simulink library "inp"  (R2021b)
settings: Solver=VariableStepAuto  StartTime=0.0  StopTime=10.0  RelTol=1e-3
undefined symbols (not defined in the file): C_TASK_5MS_S, FALSE, KINP_AcoreReadyToSlp_flg_ovrdflg, KINP_AcoreReadyToSlp_flg_ovrdval, KINP_AllowMovThd_OTA_enum_ovrdflg, KINP_AllowMovThd_OTA_enum_ovrdval, KINP_APSAngleTarget_Deg_ovrdflg, KINP_APSAngleTarget_Deg_ovrdval, KINP_APSDecReq_mps2_ovrdflg, KINP_APSDecReq_mps2_ovrdval, KINP_APSDecReqA_flg_ovrdflg, KINP_APSDecReqA_flg_ovrdval, KINP_APSDFLL_cm_ovrdflg, KINP_APSDFLL_cm_ovrdval, KINP_APSDFLR_cm_ovrdflg, KINP_APSDFLR_cm_ovrdval, KINP_APSDRLL_cm_ovrdflg, KINP_APSDRLL_cm_ovrdval, KINP_APSDRLR_cm_ovrdflg, KINP_APSDRLR_cm_ovrdval, KINP_APSExitCondition_enum_ovrdflg, KINP_APSExitCondition_enum_ovrdval, KINP_APSHWVer_enum_ovrdflg, KINP_APSHWVer_enum_ovrdval, KINP_APSProgressPCT_pct_ovrdflg, KINP_APSProgressPCT_pct_ovrdval, KINP_APSPwrReq_enum_ovrdflg, KINP_APSPwrReq_enum_ovrdval, KINP_APSReq_enum_ovrdflg, KINP_APSReq_enum_ovrdval, KINP_APSRQDisplay_enum_ovrdflg, KINP_APSRQDisplay_enum_ovrdval, KINP_APSRqEPASCtrl_flg_ovrdflg, KINP_APSRqEPASCtrl_flg_ovrdval, KINP_APSShiftPosnReq_enum_ovrdval, KINP_APSShiftPosnReq_enum_ovrflg, KINP_APSSpeedCMD_kph_ovrdval, KINP_APSSpeedCMD_kph_ovrflg, KINP_APSStaSystem_enum_ovrdflg, KINP_APSStaSystem_enum_ovrdval, KINP_APSSWVer_enum_ovrdflg, KINP_APSSWVer_enum_ovrdval, KINP_APSVMCReqA_flg_ovrdval, KINP_APSVMCReqA_flg_ovrflg, KINP_APSVRqEPASCtrl_flg_ovrdflg, KINP_APSVRqEPASCtrl_flg_ovrdval, KINP_AuxBattVolmV_mV_ovrdflg, KINP_AuxBattVolmV_mV_ovrdval, KINP_BTConnectSta_enum_ovrdflg, KINP_BTConnectSta_enum_ovrdval, KINP_CAASSta_enum_ovrdflg, KINP_CAASSta_enum_ovrdval, KINP_CAASVMCReqA_flg_ovrdval, KINP_CAASVMCReqA_flg_ovrflg, KINP_CAN1BusOff_flg_ovrdflg, KINP_CAN1BusOff_flg_ovrdval, KINP_CAN2BusOff_flg_ovrdflg, KINP_CAN2BusOff_flg_ovrdval, KINP_CAN3BusOff_flg_ovrdflg, KINP_CAN3BusOff_flg_ovrdval ... (+222)
libraries: FVT_lib x1035, hcu_lib x1
(part 26 of 33)

== system inp/INP/CAN4/SignalCheck/BodyZone_PS1 ==
  BHAL_outputs : Inport
  inp_CanValid_bus : Inport  Port=2
  BPPSEATErrorSta : FVT_lib/inp/can_signal_template  SystemSampleTime=-1  VariantActivationTime=update diagram  Latency=0  AutoFrameSizeCalculation=off
      link override defval: Value=KINP_BPPSEATErrorSta_flg_defval
      link override ovrdflg: Value=KINP_BPPSEATErrorSta_flg_ovrdflg
      link override ovrdval: Value=KINP_BPPSEATErrorSta_flg_ovrdval
  BPPSEATModeSta : FVT_lib/inp/can_signal_template  SystemSampleTime=-1  VariantActivationTime=update diagram  Latency=0  AutoFrameSizeCalculation=off
      link override defval: Value=KINP_BPPSEATModeSta_enum_defval
      link override ovrdflg: Value=KINP_BPPSEATModeSta_enum_ovrdflg
      link override ovrdval: Value=KINP_BPPSEATModeSta_enum_ovrdval
  BPPSEATVentSta : FVT_lib/inp/can_signal_template  SystemSampleTime=-1  VariantActivationTime=update diagram  Latency=0  AutoFrameSizeCalculation=off
      link override defval: Value=KINP_BPPSEATVentSta_enum_defval
      link override ovrdflg: Value=KINP_BPPSEATVentSta_enum_ovrdflg
      link override ovrdval: Value=KINP_BPPSEATVentSta_enum_ovrdval
  BPPSEATheaterSta : FVT_lib/inp/can_signal_template  SystemSampleTime=-1  VariantActivationTime=update diagram  Latency=0  AutoFrameSizeCalculation=off
      link override defval: Value=KINP_BPPSEATheaterSta_enum_defval
      link override ovrdflg: Value=KINP_BPPSEATheaterSta_enum_ovrdflg
      link override ovrdval: Value=KINP_BPPSEATheaterSta_enum_ovrdval
  BPPTGActiveSta : FVT_lib/inp/can_signal_template  SystemSampleTime=-1  VariantActivationTime=update diagram  Latency=0  AutoFrameSizeCalculation=off
      link override defval: Value=KINP_BPPTGActiveSta_enum_defval
      link override ovrdflg: Value=KINP_BPPTGActiveSta_enum_ovrdflg
      link override ovrdval: Value=KINP_BPPTGActiveSta_enum_ovrdval
  BPPTGExistSta : FVT_lib/inp/can_signal_template  SystemSampleTime=-1  VariantActivationTime=update diagram  Latency=0  AutoFrameSizeCalculation=off
      link override defval: Value=KINP_BPPTGExistSta_flg_defval
      link override ovrdflg: Value=KINP_BPPTGExistSta_flg_ovrdflg
      link override ovrdval: Value=KINP_BPPTGExistSta_flg_ovrdval
  BPPTGInsideSW1Sta : FVT_lib/inp/can_signal_template  SystemSampleTime=-1  VariantActivationTime=update diagram  Latency=0  AutoFrameSizeCalculation=off
      link override defval: Value=KINP_BPPTGInsideSW1Sta_enum_defval
      link override ovrdflg: Value=KINP_BPPTGInsideSW1Sta_enum_ovrdflg
      link override ovrdval: Value=KINP_BPPTGInsideSW1Sta_enum_ovrdval
  BPPTGInsideSW2Sta : FVT_lib/inp/can_signal_template  SystemSampleTime=-1  VariantActivationTime=update diagram  Latency=0  AutoFrameSizeCalculation=off
      link override defval: Value=KINP_BPPTGInsideSW2Sta_enum_defval
      link override ovrdflg: Value=KINP_BPPTGInsideSW2Sta_enum_ovrdflg
      link override ovrdval: Value=KINP_BPPTGInsideSW2Sta_enum_ovrdval
  BPPTGIsSetHeightSta : FVT_lib/inp/can_signal_template  SystemSampleTime=-1  VariantActivationTime=update diagram  Latency=0  AutoFrameSizeCalculation=off
      link override defval: Value=KINP_BPPTGIsSetHeightSta_flg_defval
      link override ovrdflg: Value=KINP_BPPTGIsSetHeightSta_flg_ovrdflg
      link override ovrdval: Value=KINP_BPPTGIsSetHeightSta_flg_ovrdval
  BPPTGLeftHallPosnSta : FVT_lib/inp/can_signal_template  SystemSampleTime=-1  VariantActivationTime=update diagram  Latency=0  AutoFrameSizeCalculation=off
      link override defval: Value=KINP_BPPTGLeftHallPosnSta_enum_defval
      link override ovrdflg: Value=KINP_BPPTGLeftHallPosnSta_enum_ovrdflg
      link override ovrdval: Value=KINP_BPPTGLeftHallPosnSta_enum_ovrdval
  BPPTGOpenRatioSta : FVT_lib/inp/can_signal_template  SystemSampleTime=-1  VariantActivationTime=update diagram  Latency=0  AutoFrameSizeCalculation=off
      link override defval: Value=KINP_BPPTGOpenRatioSta_pct_defval
      link override ovrdflg: Value=KINP_BPPTGOpenRatioSta_pct_ovrdflg
      link override ovrdval: Value=KINP_BPPTGOpenRatioSta_pct_ovrdval
  BPPTGRDILCmd : FVT_lib/inp/can_signal_template  SystemSampleTime=-1  VariantActivationTime=update diagram  Latency=0  AutoFrameSizeCalculation=off
      link override defval: Value=KINP_BPPTGRDILCmd_enum_defval
      link override ovrdflg: Value=KINP_BPPTGRDILCmd_enum_ovrdflg
      link override ovrdval: Value=KINP_BPPTGRDILCmd_enum_ovrdval
  BPPTGSysSta : FVT_lib/inp/can_signal_template  SystemSampleTime=-1  VariantActivationTime=update diagram  Latency=0  AutoFrameSizeCalculation=off
      link override defval: Value=KINP_BPPTGSysSta_enum_defval
      link override ovrdflg: Value=KINP_BPPTGSysSta_enum_ovrdflg
      link override ovrdval: Value=KINP_BPPTGSysSta_enum_ovrdval
  Terminator_{1..13} (13 alike) : Terminator
  True_VHAL_BPPSEATErrorSta_flg : Constant  Value=TRUE  OutDataTypeStr=boolean
  True_VHAL_BPPSEATModeSta_enum : Constant  Value=TRUE  OutDataTypeStr=boolean
  True_VHAL_BPPSEATVentSta_enum : Constant  Value=TRUE  OutDataTypeStr=boolean
  True_VHAL_BPPSEATheaterSta_enum : Constant  Value=TRUE  OutDataTypeStr=boolean
  True_VHAL_BPPTGActiveSta_enum : Constant  Value=TRUE  OutDataTypeStr=boolean
  True_VHAL_BPPTGExistSta_flg : Constant  Value=TRUE  OutDataTypeStr=boolean
  True_VHAL_BPPTGInsideSW1Sta_enum : Constant  Value=TRUE  OutDataTypeStr=boolean
  True_VHAL_BPPTGInsideSW2Sta_enum : Constant  Value=TRUE  OutDataTypeStr=boolean
  True_VHAL_BPPTGIsSetHeightSta_flg : Constant  Value=TRUE  OutDataTypeStr=boolean
  True_VHAL_BPPTGLeftHallPosnSta_enum : Constant  Value=TRUE  OutDataTypeStr=boolean
  True_VHAL_BPPTGOpenRatioSta_pct : Constant  Value=TRUE  OutDataTypeStr=boolean
  True_VHAL_BPPTGRDILCmd_enum : Constant  Value=TRUE  OutDataTypeStr=boolean
  True_VHAL_BPPTGSysSta_enum : Constant  Value=TRUE  OutDataTypeStr=boolean
  slr1_{1..13} (13 alike) : BusSelector  OutputSignals=VINP_CANMsgValidBodyZonePS1_flg
  slr_VHAL_BPPSEATErrorSta_flg : BusSelector  OutputSignals=VHAL_BPPSEATErrorSta_flg
  slr_VHAL_BPPSEATModeSta_enum : BusSelector  OutputSignals=VHAL_BPPSEATModeSta_enum
  slr_VHAL_BPPSEATVentSta_enum : BusSelector  OutputSignals=VHAL_BPPSEATVentSta_enum
  slr_VHAL_BPPSEATheaterSta_enum : BusSelector  OutputSignals=VHAL_BPPSEATheaterSta_enum
  slr_VHAL_BPPTGActiveSta_enum : BusSelector  OutputSignals=VHAL_BPPTGActiveSta_enum
  slr_VHAL_BPPTGExistSta_flg : BusSelector  OutputSignals=VHAL_BPPTGExistSta_flg
  slr_VHAL_BPPTGInsideSW1Sta_enum : BusSelector  OutputSignals=VHAL_BPPTGInsideSW1Sta_enum
  slr_VHAL_BPPTGInsideSW2Sta_enum : BusSelector  OutputSignals=VHAL_BPPTGInsideSW2Sta_enum
  slr_VHAL_BPPTGIsSetHeightSta_flg : BusSelector  OutputSignals=VHAL_BPPTGIsSetHeightSta_flg
  slr_VHAL_BPPTGLeftHallPosnSta_enum : BusSelector  OutputSignals=VHAL_BPPTGLeftHallPosnSta_enum
  slr_VHAL_BPPTGOpenRatioSta_pct : BusSelector  OutputSignals=VHAL_BPPTGOpenRatioSta_pct
  slr_VHAL_BPPTGRDILCmd_enum : BusSelector  OutputSignals=VHAL_BPPTGRDILCmd_enum
  slr_VHAL_BPPTGSysSta_enum : BusSelector  OutputSignals=VHAL_BPPTGSysSta_enum
  VINP_BPPSEATErrorSta_flg : Outport
  VINP_BPPSEATModeSta_enum : Outport  Port=2
  VINP_BPPSEATVentSta_enum : Outport  Port=3
  VINP_BPPSEATheaterSta_enum : Outport  Port=4
  VINP_BPPTGActiveSta_enum : Outport  Port=5
  VINP_BPPTGExistSta_flg : Outport  Port=6
  VINP_BPPTGInsideSW1Sta_enum : Outport  Port=7
  VINP_BPPTGInsideSW2Sta_enum : Outport  Port=8
  VINP_BPPTGIsSetHeightSta_flg : Outport  Port=9
  VINP_BPPTGLeftHallPosnSta_enum : Outport  Port=10
  VINP_BPPTGOpenRatioSta_pct : Outport  Port=11
  VINP_BPPTGRDILCmd_enum : Outport  Port=12
  VINP_BPPTGSysSta_enum : Outport  Port=13
  wires:
  BHAL_outputs/1 -> [BHAL_outputs]
  inp_CanValid_bus/1 -> [inp_CanValid_bus]
  [BHAL_outputs] -> slr_VHAL_BPPSEATErrorSta_flg/1
  slr_VHAL_BPPSEATErrorSta_flg/1 -> BPPSEATErrorSta/1  "<VHAL_BPPSEATErrorSta_flg>"
  True_VHAL_BPPSEATErrorSta_flg/1 -> BPPSEATErrorSta/2
  [inp_CanValid_bus] -> slr1_1/1
  slr1_1/1 -> BPPSEATErrorSta/3  "<VINP_CANMsgValidBodyZonePS1_flg>"
  BPPSEATErrorSta/1 -> VINP_BPPSEATErrorSta_flg/1  "VINP_BPPSEATErrorSta_flg"
  BPPSEATErrorSta/2 -> Terminator_1/1
  [BHAL_outputs] -> slr_VHAL_BPPSEATModeSta_enum/1
  slr_VHAL_BPPSEATModeSta_enum/1 -> BPPSEATModeSta/1  "<VHAL_BPPSEATModeSta_enum>"
  True_VHAL_BPPSEATModeSta_enum/1 -> BPPSEATModeSta/2
  [inp_CanValid_bus] -> slr1_2/1
  slr1_2/1 -> BPPSEATModeSta/3  "<VINP_CANMsgValidBodyZonePS1_flg>"
  BPPSEATModeSta/1 -> VINP_BPPSEATModeSta_enum/1  "VINP_BPPSEATModeSta_enum"
  BPPSEATModeSta/2 -> Terminator_2/1
  [BHAL_outputs] -> slr_VHAL_BPPSEATVentSta_enum/1
  slr_VHAL_BPPSEATVentSta_enum/1 -> BPPSEATVentSta/1  "<VHAL_BPPSEATVentSta_enum>"
  True_VHAL_BPPSEATVentSta_enum/1 -> BPPSEATVentSta/2
  [inp_CanValid_bus] -> slr1_3/1
  slr1_3/1 -> BPPSEATVentSta/3  "<VINP_CANMsgValidBodyZonePS1_flg>"
  BPPSEATVentSta/1 -> VINP_BPPSEATVentSta_enum/1  "VINP_BPPSEATVentSta_enum"
  BPPSEATVentSta/2 -> Terminator_3/1
  [BHAL_outputs] -> slr_VHAL_BPPSEATheaterSta_enum/1
  slr_VHAL_BPPSEATheaterSta_enum/1 -> BPPSEATheaterSta/1  "<VHAL_BPPSEATheaterSta_enum>"
  True_VHAL_BPPSEATheaterSta_enum/1 -> BPPSEATheaterSta/2
  [inp_CanValid_bus] -> slr1_4/1
  slr1_4/1 -> BPPSEATheaterSta/3  "<VINP_CANMsgValidBodyZonePS1_flg>"
  BPPSEATheaterSta/1 -> VINP_BPPSEATheaterSta_enum/1  "VINP_BPPSEATheaterSta_enum"
  BPPSEATheaterSta/2 -> Terminator_4/1
  [BHAL_outputs] -> slr_VHAL_BPPTGActiveSta_enum/1
  slr_VHAL_BPPTGActiveSta_enum/1 -> BPPTGActiveSta/1  "<VHAL_BPPTGActiveSta_enum>"
  True_VHAL_BPPTGActiveSta_enum/1 -> BPPTGActiveSta/2
  [inp_CanValid_bus] -> slr1_5/1
  slr1_5/1 -> BPPTGActiveSta/3  "<VINP_CANMsgValidBodyZonePS1_flg>"
  BPPTGActiveSta/1 -> VINP_BPPTGActiveSta_enum/1  "VINP_BPPTGActiveSta_enum"
  BPPTGActiveSta/2 -> Terminator_5/1
  [BHAL_outputs] -> slr_VHAL_BPPTGExistSta_flg/1
  slr_VHAL_BPPTGExistSta_flg/1 -> BPPTGExistSta/1  "<VHAL_BPPTGExistSta_flg>"
  True_VHAL_BPPTGExistSta_flg/1 -> BPPTGExistSta/2
  [inp_CanValid_bus] -> slr1_6/1
  slr1_6/1 -> BPPTGExistSta/3  "<VINP_CANMsgValidBodyZonePS1_flg>"
  BPPTGExistSta/1 -> VINP_BPPTGExistSta_flg/1  "VINP_BPPTGExistSta_flg"
  BPPTGExistSta/2 -> Terminator_6/1
  [BHAL_outputs] -> slr_VHAL_BPPTGInsideSW1Sta_enum/1
  slr_VHAL_BPPTGInsideSW1Sta_enum/1 -> BPPTGInsideSW1Sta/1  "<VHAL_BPPTGInsideSW1Sta_enum>"
  True_VHAL_BPPTGInsideSW1Sta_enum/1 -> BPPTGInsideSW1Sta/2
  [inp_CanValid_bus] -> slr1_7/1
  slr1_7/1 -> BPPTGInsideSW1Sta/3  "<VINP_CANMsgValidBodyZonePS1_flg>"
  BPPTGInsideSW1Sta/1 -> VINP_BPPTGInsideSW1Sta_enum/1  "VINP_BPPTGInsideSW1Sta_enum"
  BPPTGInsideSW1Sta/2 -> Terminator_7/1
  [BHAL_outputs] -> slr_VHAL_BPPTGInsideSW2Sta_enum/1
  slr_VHAL_BPPTGInsideSW2Sta_enum/1 -> BPPTGInsideSW2Sta/1  "<VHAL_BPPTGInsideSW2Sta_enum>"
  True_VHAL_BPPTGInsideSW2Sta_enum/1 -> BPPTGInsideSW2Sta/2
  [inp_CanValid_bus] -> slr1_8/1
  slr1_8/1 -> BPPTGInsideSW2Sta/3  "<VINP_CANMsgValidBodyZonePS1_flg>"
  BPPTGInsideSW2Sta/1 -> VINP_BPPTGInsideSW2Sta_enum/1  "VINP_BPPTGInsideSW2Sta_enum"
  BPPTGInsideSW2Sta/2 -> Terminator_8/1
  [BHAL_outputs] -> slr_VHAL_BPPTGIsSetHeightSta_flg/1
  slr_VHAL_BPPTGIsSetHeightSta_flg/1 -> BPPTGIsSetHeightSta/1  "<VHAL_BPPTGIsSetHeightSta_flg>"
  True_VHAL_BPPTGIsSetHeightSta_flg/1 -> BPPTGIsSetHeightSta/2
  [inp_CanValid_bus] -> slr1_9/1
  slr1_9/1 -> BPPTGIsSetHeightSta/3  "<VINP_CANMsgValidBodyZonePS1_flg>"
  BPPTGIsSetHeightSta/1 -> VINP_BPPTGIsSetHeightSta_flg/1  "VINP_BPPTGIsSetHeightSta_flg"
  BPPTGIsSetHeightSta/2 -> Terminator_9/1
  [BHAL_outputs] -> slr_VHAL_BPPTGLeftHallPosnSta_enum/1
  slr_VHAL_BPPTGLeftHallPosnSta_enum/1 -> BPPTGLeftHallPosnSta/1  "<VHAL_BPPTGLeftHallPosnSta_enum>"
  True_VHAL_BPPTGLeftHallPosnSta_enum/1 -> BPPTGLeftHallPosnSta/2
  [inp_CanValid_bus] -> slr1_10/1
  slr1_10/1 -> BPPTGLeftHallPosnSta/3  "<VINP_CANMsgValidBodyZonePS1_flg>"
  BPPTGLeftHallPosnSta/1 -> VINP_BPPTGLeftHallPosnSta_enum/1  "VINP_BPPTGLeftHallPosnSta_enum"
  BPPTGLeftHallPosnSta/2 -> Terminator_10/1
  [BHAL_outputs] -> slr_VHAL_BPPTGOpenRatioSta_pct/1
  slr_VHAL_BPPTGOpenRatioSta_pct/1 -> BPPTGOpenRatioSta/1  "<VHAL_BPPTGOpenRatioSta_pct>"
  True_VHAL_BPPTGOpenRatioSta_pct/1 -> BPPTGOpenRatioSta/2
  [inp_CanValid_bus] -> slr1_11/1
  slr1_11/1 -> BPPTGOpenRatioSta/3  "<VINP_CANMsgValidBodyZonePS1_flg>"
  BPPTGOpenRatioSta/1 -> VINP_BPPTGOpenRatioSta_pct/1  "VINP_BPPTGOpenRatioSta_pct"
  BPPTGOpenRatioSta/2 -> Terminator_11/1
  [BHAL_outputs] -> slr_VHAL_BPPTGRDILCmd_enum/1
  slr_VHAL_BPPTGRDILCmd_enum/1 -> BPPTGRDILCmd/1  "<VHAL_BPPTGRDILCmd_enum>"
  True_VHAL_BPPTGRDILCmd_enum/1 -> BPPTGRDILCmd/2
  [inp_CanValid_bus] -> slr1_12/1
  slr1_12/1 -> BPPTGRDILCmd/3  "<VINP_CANMsgValidBodyZonePS1_flg>"
  BPPTGRDILCmd/1 -> VINP_BPPTGRDILCmd_enum/1  "VINP_BPPTGRDILCmd_enum"
  BPPTGRDILCmd/2 -> Terminator_12/1
  [BHAL_outputs] -> slr_VHAL_BPPTGSysSta_enum/1
  slr_VHAL_BPPTGSysSta_enum/1 -> BPPTGSysSta/1  "<VHAL_BPPTGSysSta_enum>"
  True_VHAL_BPPTGSysSta_enum/1 -> BPPTGSysSta/2
  [inp_CanValid_bus] -> slr1_13/1
  slr1_13/1 -> BPPTGSysSta/3  "<VINP_CANMsgValidBodyZonePS1_flg>"
  BPPTGSysSta/1 -> VINP_BPPTGSysSta_enum/1  "VINP_BPPTGSysSta_enum"
  BPPTGSysSta/2 -> Terminator_13/1

== system inp/INP/CAN4/SignalCheck/BodyZone_PS2 ==
  BHAL_outputs : Inport
  inp_CanValid_bus : Inport  Port=2
  BPAPMWinFOpenedSta : FVT_lib/inp/can_signal_template  SystemSampleTime=-1  VariantActivationTime=update diagram  Latency=0  AutoFrameSizeCalculation=off
      link override defval: Value=KINP_BPAPMWinFOpenedSta_pct_defval
      link override ovrdflg: Value=KINP_BPAPMWinFOpenedSta_pct_ovrdflg
      link override ovrdval: Value=KINP_BPAPMWinFOpenedSta_pct_ovrdval
  BPAPMWinROpenedSta : FVT_lib/inp/can_signal_template  SystemSampleTime=-1  VariantActivationTime=update diagram  Latency=0  AutoFrameSizeCalculation=off
      link override defval: Value=KINP_BPAPMWinROpenedSta_pct_defval
      link override ovrdflg: Value=KINP_BPAPMWinROpenedSta_pct_ovrdflg
      link override ovrdval: Value=KINP_BPAPMWinROpenedSta_pct_ovrdval
  BPDoorFHandleCloseSta : FVT_lib/inp/can_signal_template  SystemSampleTime=-1  VariantActivationTime=update diagram  Latency=0  AutoFrameSizeCalculation=off
      link override defval: Value=KINP_BPDoorFHandleCloseSta_flg_defval
      link override ovrdflg: Value=KINP_BPDoorFHandleCloseSta_flg_ovrdflg
      link override ovrdval: Value=KINP_BPDoorFHandleCloseSta_flg_ovrdval
  BPDoorRHandleCloseSta : FVT_lib/inp/can_signal_template  SystemSampleTime=-1  VariantActivationTime=update diagram  Latency=0  AutoFrameSizeCalculation=off
      link override defval: Value=KINP_BPDoorRHandleCloseSta_flg_defval
      link override ovrdflg: Value=KINP_BPDoorRHandleCloseSta_flg_ovrdflg
      link override ovrdval: Value=KINP_BPDoorRHandleCloseSta_flg_ovrdval
  BPSEATLVentSta : FVT_lib/inp/can_signal_template  SystemSampleTime=-1  VariantActivationTime=update diagram  Latency=0  AutoFrameSizeCalculation=off
      link override defval: Value=KINP_BPSEATLVentSta_enum_defval
      link override ovrdflg: Value=KINP_BPSEATLVentSta_enum_ovrdflg
      link override ovrdval: Value=KINP_BPSEATLVentSta_enum_ovrdval
  BPSEATMLVentSta : FVT_lib/inp/can_signal_template  SystemSampleTime=-1  VariantActivationTime=update diagram  Latency=0  AutoFrameSizeCalculation=off
      link override defval: Value=KINP_BPSEATMLVentSta_enum_defval
      link override ovrdflg: Value=KINP_BPSEATMLVentSta_enum_ovrdflg
      link override ovrdval: Value=KINP_BPSEATMLVentSta_enum_ovrdval
  BPSEATMRVentSta : FVT_lib/inp/can_signal_template  SystemSampleTime=-1  VariantActivationTime=update diagram  Latency=0  AutoFrameSizeCalculation=off
      link override defval: Value=KINP_BPSEATMRVentSta_enum_defval
      link override ovrdflg: Value=KINP_BPSEATMRVentSta_enum_ovrdflg
      link override ovrdval: Value=KINP_BPSEATMRVentSta_enum_ovrdval
  BPSEATRVentSta : FVT_lib/inp/can_signal_template  SystemSampleTime=-1  VariantActivationTime=update diagram  Latency=0  AutoFrameSizeCalculation=off
      link override defval: Value=KINP_BPSEATRVentSta_enum_defval
      link override ovrdflg: Value=KINP_BPSEATRVentSta_enum_ovrdflg
      link override ovrdval: Value=KINP_BPSEATRVentSta_enum_ovrdval
  Terminator_{1..8} (8 alike) : Terminator
  True_VHAL_BPAPMWinFOpenedSta_pct : Constant  Value=TRUE  OutDataTypeStr=boolean
  True_VHAL_BPAPMWinROpenedSta_pct : Constant  Value=TRUE  OutDataTypeStr=boolean
  True_VHAL_BPDoorFHandleCloseSta_flg : Constant  Value=TRUE  OutDataTypeStr=boolean
  True_VHAL_BPDoorRHandleCloseSta_flg : Constant  Value=TRUE  OutDataTypeStr=boolean
  True_VHAL_BPSEATLVentSta_enum : Constant  Value=TRUE  OutDataTypeStr=boolean
  True_VHAL_BPSEATMLVentSta_enum : Constant  Value=TRUE  OutDataTypeStr=boolean
  True_VHAL_BPSEATMRVentSta_enum : Constant  Value=TRUE  OutDataTypeStr=boolean
  True_VHAL_BPSEATRVentSta_enum : Constant  Value=TRUE  OutDataTypeStr=boolean
  slr1_{1..8} (8 alike) : BusSelector  OutputSignals=VINP_CANMsgValidBodyZonePS2_flg
  slr_VHAL_BPAPMWinFOpenedSta_pct : BusSelector  OutputSignals=VHAL_BPAPMWinFOpenedSta_pct
  slr_VHAL_BPAPMWinROpenedSta_pct : BusSelector  OutputSignals=VHAL_BPAPMWinROpenedSta_pct
  slr_VHAL_BPDoorFHandleCloseSta_flg : BusSelector  OutputSignals=VHAL_BPDoorFHandleCloseSta_flg
  slr_VHAL_BPDoorRHandleCloseSta_flg : BusSelector  OutputSignals=VHAL_BPDoorRHandleCloseSta_flg
  slr_VHAL_BPSEATLVentSta_enum : BusSelector  OutputSignals=VHAL_BPSEATLVentSta_enum
  slr_VHAL_BPSEATMLVentSta_enum : BusSelector  OutputSignals=VHAL_BPSEATMLVentSta_enum
  slr_VHAL_BPSEATMRVentSta_enum : BusSelector  OutputSignals=VHAL_BPSEATMRVentSta_enum
  slr_VHAL_BPSEATRVentSta_enum : BusSelector  OutputSignals=VHAL_BPSEATRVentSta_enum
  VINP_BPAPMWinFOpenedSta_pct : Outport
  VINP_BPAPMWinROpenedSta_pct : Outport  Port=2
  VINP_BPDoorFHandleCloseSta_flg : Outport  Port=3
  VINP_BPDoorRHandleCloseSta_flg : Outport  Port=4
  VINP_BPSEATLVentSta_enum : Outport  Port=5
  VINP_BPSEATMLVentSta_enum : Outport  Port=6
  VINP_BPSEATMRVentSta_enum : Outport  Port=7
  VINP_BPSEATRVentSta_enum : Outport  Port=8
  wires:
  BHAL_outputs/1 -> [BHAL_outputs]
  inp_CanValid_bus/1 -> [inp_CanValid_bus]
  [BHAL_outputs] -> slr_VHAL_BPAPMWinFOpenedSta_pct/1
  slr_VHAL_BPAPMWinFOpenedSta_pct/1 -> BPAPMWinFOpenedSta/1  "<VHAL_BPAPMWinFOpenedSta_pct>"
  True_VHAL_BPAPMWinFOpenedSta_pct/1 -> BPAPMWinFOpenedSta/2
  [inp_CanValid_bus] -> slr1_1/1
  slr1_1/1 -> BPAPMWinFOpenedSta/3  "<VINP_CANMsgValidBodyZonePS2_flg>"
  BPAPMWinFOpenedSta/1 -> VINP_BPAPMWinFOpenedSta_pct/1  "VINP_BPAPMWinFOpenedSta_pct"
  BPAPMWinFOpenedSta/2 -> Terminator_1/1
  [BHAL_outputs] -> slr_VHAL_BPAPMWinROpenedSta_pct/1
  slr_VHAL_BPAPMWinROpenedSta_pct/1 -> BPAPMWinROpenedSta/1  "<VHAL_BPAPMWinROpenedSta_pct>"
  True_VHAL_BPAPMWinROpenedSta_pct/1 -> BPAPMWinROpenedSta/2
  [inp_CanValid_bus] -> slr1_2/1
  slr1_2/1 -> BPAPMWinROpenedSta/3  "<VINP_CANMsgValidBodyZonePS2_flg>"
  BPAPMWinROpenedSta/1 -> VINP_BPAPMWinROpenedSta_pct/1  "VINP_BPAPMWinROpenedSta_pct"
  BPAPMWinROpenedSta/2 -> Terminator_2/1
  [BHAL_outputs] -> slr_VHAL_BPDoorFHandleCloseSta_flg/1
  slr_VHAL_BPDoorFHandleCloseSta_flg/1 -> BPDoorFHandleCloseSta/1  "<VHAL_BPDoorFHandleCloseSta_flg>"
  True_VHAL_BPDoorFHandleCloseSta_flg/1 -> BPDoorFHandleCloseSta/2
  [inp_CanValid_bus] -> slr1_3/1
  slr1_3/1 -> BPDoorFHandleCloseSta/3  "<VINP_CANMsgValidBodyZonePS2_flg>"
  BPDoorFHandleCloseSta/1 -> VINP_BPDoorFHandleCloseSta_flg/1  "VINP_BPDoorFHandleCloseSta_flg"
  BPDoorFHandleCloseSta/2 -> Terminator_3/1
  [BHAL_outputs] -> slr_VHAL_BPDoorRHandleCloseSta_flg/1
  slr_VHAL_BPDoorRHandleCloseSta_flg/1 -> BPDoorRHandleCloseSta/1  "<VHAL_BPDoorRHandleCloseSta_flg>"
  True_VHAL_BPDoorRHandleCloseSta_flg/1 -> BPDoorRHandleCloseSta/2
  [inp_CanValid_bus] -> slr1_4/1
  slr1_4/1 -> BPDoorRHandleCloseSta/3  "<VINP_CANMsgValidBodyZonePS2_flg>"
  BPDoorRHandleCloseSta/1 -> VINP_BPDoorRHandleCloseSta_flg/1  "VINP_BPDoorRHandleCloseSta_flg"
  BPDoorRHandleCloseSta/2 -> Terminator_4/1
  [BHAL_outputs] -> slr_VHAL_BPSEATLVentSta_enum/1
  slr_VHAL_BPSEATLVentSta_enum/1 -> BPSEATLVentSta/1  "<VHAL_BPSEATLVentSta_enum>"
  True_VHAL_BPSEATLVentSta_enum/1 -> BPSEATLVentSta/2
  [inp_CanValid_bus] -> slr1_5/1
  slr1_5/1 -> BPSEATLVentSta/3  "<VINP_CANMsgValidBodyZonePS2_flg>"
  BPSEATLVentSta/1 -> VINP_BPSEATLVentSta_enum/1  "VINP_BPSEATLVentSta_enum"
  BPSEATLVentSta/2 -> Terminator_5/1
  [BHAL_outputs] -> slr_VHAL_BPSEATMLVentSta_enum/1
  slr_VHAL_BPSEATMLVentSta_enum/1 -> BPSEATMLVentSta/1  "<VHAL_BPSEATMLVentSta_enum>"
  True_VHAL_BPSEATMLVentSta_enum/1 -> BPSEATMLVentSta/2
  [inp_CanValid_bus] -> slr1_6/1
  slr1_6/1 -> BPSEATMLVentSta/3  "<VINP_CANMsgValidBodyZonePS2_flg>"
  BPSEATMLVentSta/1 -> VINP_BPSEATMLVentSta_enum/1  "VINP_BPSEATMLVentSta_enum"
  BPSEATMLVentSta/2 -> Terminator_6/1
  [BHAL_outputs] -> slr_VHAL_BPSEATMRVentSta_enum/1
  slr_VHAL_BPSEATMRVentSta_enum/1 -> BPSEATMRVentSta/1  "<VHAL_BPSEATMRVentSta_enum>"
  True_VHAL_BPSEATMRVentSta_enum/1 -> BPSEATMRVentSta/2
  [inp_CanValid_bus] -> slr1_7/1
  slr1_7/1 -> BPSEATMRVentSta/3  "<VINP_CANMsgValidBodyZonePS2_flg>"
  BPSEATMRVentSta/1 -> VINP_BPSEATMRVentSta_enum/1  "VINP_BPSEATMRVentSta_enum"
  BPSEATMRVentSta/2 -> Terminator_7/1
  [BHAL_outputs] -> slr_VHAL_BPSEATRVentSta_enum/1
  slr_VHAL_BPSEATRVentSta_enum/1 -> BPSEATRVentSta/1  "<VHAL_BPSEATRVentSta_enum>"
  True_VHAL_BPSEATRVentSta_enum/1 -> BPSEATRVentSta/2
  [inp_CanValid_bus] -> slr1_8/1
  slr1_8/1 -> BPSEATRVentSta/3  "<VINP_CANMsgValidBodyZonePS2_flg>"
  BPSEATRVentSta/1 -> VINP_BPSEATRVentSta_enum/1  "VINP_BPSEATRVentSta_enum"
  BPSEATRVentSta/2 -> Terminator_8/1

== system inp/INP/CAN4/SignalCheck/DKC1 ==
  BHAL_outputs : Inport
  inp_CanValid_bus : Inport  Port=2
  DKCKeyNumSta : FVT_lib/inp/can_signal_template  SystemSampleTime=-1  VariantActivationTime=update diagram  Latency=0  AutoFrameSizeCalculation=off
      link override defval: Value=KINP_DKCKeyNumSta_enum_defval
      link override ovrdflg: Value=KINP_DKCKeyNumSta_enum_ovrdflg
      link override ovrdval: Value=KINP_DKCKeyNumSta_enum_ovrdval
  DKCKeyTypeSta : FVT_lib/inp/can_signal_template  SystemSampleTime=-1  VariantActivationTime=update diagram  Latency=0  AutoFrameSizeCalculation=off
      link override defval: Value=KINP_DKCKeyTypeSta_enum_defval
      link override ovrdflg: Value=KINP_DKCKeyTypeSta_enum_ovrdflg
      link override ovrdval: Value=KINP_DKCKeyTypeSta_enum_ovrdval
  DKCPDkeyAreaRAPSSta : FVT_lib/inp/can_signal_template  SystemSampleTime=-1  VariantActivationTime=update diagram  Latency=0  AutoFrameSizeCalculation=off
      link override defval: Value=KINP_DKCPDkeyAreaRAPSSta_enum_defval
      link override ovrdflg: Value=KINP_DKCPDkeyAreaRAPSSta_enum_ovrdflg
      link override ovrdval: Value=KINP_DKCPDkeyAreaRAPSSta_enum_ovrdval
  DKCParkingModeCmd : FVT_lib/inp/can_signal_template  SystemSampleTime=-1  VariantActivationTime=update diagram  Latency=0  AutoFrameSizeCalculation=off
      link override defval: Value=KINP_DKCParkingModeCmd_enum_defval
      link override ovrdflg: Value=KINP_DKCParkingModeCmd_enum_ovrdflg
      link override ovrdval: Value=KINP_DKCParkingModeCmd_enum_ovrdval
  DKCReVehData : FVT_lib/inp/can_signal_template  SystemSampleTime=-1  VariantActivationTime=update diagram  Latency=0  AutoFrameSizeCalculation=off
      link override defval: Value=KINP_DKCReVehData_enum_defval
      link override ovrdflg: Value=KINP_DKCReVehData_enum_ovrdflg
      link override ovrdval: Value=KINP_DKCReVehData_enum_ovrdval
  PCommandToBCM : FVT_lib/inp/can_signal_template  SystemSampleTime=-1  VariantActivationTime=update diagram  Latency=0  AutoFrameSizeCalculation=off
      link override defval: Value=KINP_PCommandToBCM_enum_defval
      link override ovrdflg: Value=KINP_PCommandToBCM_enum_ovrdflg
      link override ovrdval: Value=KINP_PCommandToBCM_enum_ovrdval
  PCommandToPTG : FVT_lib/inp/can_signal_template  SystemSampleTime=-1  VariantActivationTime=update diagram  Latency=0  AutoFrameSizeCalculation=off
      link override defval: Value=KINP_PCommandToPTG_enum_defval
      link override ovrdflg: Value=KINP_PCommandToPTG_enum_ovrdflg
      link override ovrdval: Value=KINP_PCommandToPTG_enum_ovrdval
  PDKeyAreaLockUnlock : FVT_lib/inp/can_signal_template  SystemSampleTime=-1  VariantActivationTime=update diagram  Latency=0  AutoFrameSizeCalculation=off
      link override defval: Value=KINP_PDKeyAreaLockUnlock_enum_defval
      link override ovrdflg: Value=KINP_PDKeyAreaLockUnlock_enum_ovrdflg
      link override ovrdval: Value=KINP_PDKeyAreaLockUnlock_enum_ovrdval
  PDKeyAreaPS : FVT_lib/inp/can_signal_template  SystemSampleTime=-1  VariantActivationTime=update diagram  Latency=0  AutoFrameSizeCalculation=off
      link override defval: Value=KINP_PDKeyAreaPS_enum_defval
      link override ovrdflg: Value=KINP_PDKeyAreaPS_enum_ovrdflg
      link override ovrdval: Value=KINP_PDKeyAreaPS_enum_ovrdval
  PDKeyAreaPTG : FVT_lib/inp/can_signal_template  SystemSampleTime=-1  VariantActivationTime=update diagram  Latency=0  AutoFrameSizeCalculation=off
      link override defval: Value=KINP_PDKeyAreaPTG_enum_defval
      link override ovrdflg: Value=KINP_PDKeyAreaPTG_enum_ovrdflg
      link override ovrdval: Value=KINP_PDKeyAreaPTG_enum_ovrdval
  PDKeyWelcome : FVT_lib/inp/can_signal_template  SystemSampleTime=-1  VariantActivationTime=update diagram  Latency=0  AutoFrameSizeCalculation=off
      link override defval: Value=KINP_PDKeyWelcome_enum_defval
      link override ovrdflg: Value=KINP_PDKeyWelcome_enum_ovrdflg
      link override ovrdval: Value=KINP_PDKeyWelcome_enum_ovrdval
  PDkeyShowIVI : FVT_lib/inp/can_signal_template  SystemSampleTime=-1  VariantActivationTime=update diagram  Latency=0  AutoFrameSizeCalculation=off
      link override defval: Value=KINP_PDkeyShowIVI_enum_defval
      link override ovrdflg: Value=KINP_PDkeyShowIVI_enum_ovrdflg
      link override ovrdval: Value=KINP_PDkeyShowIVI_enum_ovrdval
  PKeyMiss : FVT_lib/inp/can_signal_template  SystemSampleTime=-1  VariantActivationTime=update diagram  Latency=0  AutoFrameSizeCalculation=off
      link override defval: Value=KINP_PKeyMiss_flg_defval
      link override ovrdflg: Value=KINP_PKeyMiss_flg_ovrdflg
      link override ovrdval: Value=KINP_PKeyMiss_flg_ovrdval
  PKeyMode : FVT_lib/inp/can_signal_template  SystemSampleTime=-1  VariantActivationTime=update diagram  Latency=0  AutoFrameSizeCalculation=off
      link override defval: Value=KINP_PKeyMode_enum_defval
      link override ovrdflg: Value=KINP_PKeyMode_enum_ovrdflg
      link override ovrdval: Value=KINP_PKeyMode_enum_ovrdval
  PUIDLowPower : FVT_lib/inp/can_signal_template  SystemSampleTime=-1  VariantActivationTime=update diagram  Latency=0  AutoFrameSizeCalculation=off
      link override defval: Value=KINP_PUIDLowPower_flg_defval
      link override ovrdflg: Value=KINP_PUIDLowPower_flg_ovrdflg
      link override ovrdval: Value=KINP_PUIDLowPower_flg_ovrdval
  Terminator_{1..15} (15 alike) : Terminator
  True_VHAL_DKCKeyNumSta_enum : Constant  Value=TRUE  OutDataTypeStr=boolean
  True_VHAL_DKCKeyTypeSta_enum : Constant  Value=TRUE  OutDataTypeStr=boolean
  True_VHAL_DKCPDkeyAreaRAPSSta_enum : Constant  Value=TRUE  OutDataTypeStr=boolean
  True_VHAL_DKCParkingModeCmd_enum : Constant  Value=TRUE  OutDataTypeStr=boolean
  True_VHAL_DKCReVehData_enum : Constant  Value=TRUE  OutDataTypeStr=boolean
  True_VHAL_PCommandToBCM_enum : Constant  Value=TRUE  OutDataTypeStr=boolean
  True_VHAL_PCommandToPTG_enum : Constant  Value=TRUE  OutDataTypeStr=boolean
  True_VHAL_PDKeyAreaLockUnlock_enum : Constant  Value=TRUE  OutDataTypeStr=boolean
  True_VHAL_PDKeyAreaPS_enum : Constant  Value=TRUE  OutDataTypeStr=boolean
  True_VHAL_PDKeyAreaPTG_enum : Constant  Value=TRUE  OutDataTypeStr=boolean
  True_VHAL_PDKeyWelcome_enum : Constant  Value=TRUE  OutDataTypeStr=boolean
  True_VHAL_PDkeyShowIVI_enum : Constant  Value=TRUE  OutDataTypeStr=boolean
  True_VHAL_PKeyMiss_flg : Constant  Value=TRUE  OutDataTypeStr=boolean
  True_VHAL_PKeyMode_enum : Constant  Value=TRUE  OutDataTypeStr=boolean
  True_VHAL_PUIDLowPower_flg : Constant  Value=TRUE  OutDataTypeStr=boolean
  slr1_{1..15} (15 alike) : BusSelector  OutputSignals=VINP_CANMsgValidDKC1_flg
  slr_VHAL_DKCKeyNumSta_enum : BusSelector  OutputSignals=VHAL_DKCKeyNumSta_enum
  slr_VHAL_DKCKeyTypeSta_enum : BusSelector  OutputSignals=VHAL_DKCKeyTypeSta_enum
  slr_VHAL_DKCPDkeyAreaRAPSSta_enum : BusSelector  OutputSignals=VHAL_DKCPDkeyAreaRAPSSta_enum
  slr_VHAL_DKCParkingModeCmd_enum : BusSelector  OutputSignals=VHAL_DKCParkingModeCmd_enum
  slr_VHAL_DKCReVehData_enum : BusSelector  OutputSignals=VHAL_DKCReVehData_enum
  slr_VHAL_PCommandToBCM_enum : BusSelector  OutputSignals=VHAL_PCommandToBCM_enum
  slr_VHAL_PCommandToPTG_enum : BusSelector  OutputSignals=VHAL_PCommandToPTG_enum
  slr_VHAL_PDKeyAreaLockUnlock_enum : BusSelector  OutputSignals=VHAL_PDKeyAreaLockUnlock_enum
  slr_VHAL_PDKeyAreaPS_enum : BusSelector  OutputSignals=VHAL_PDKeyAreaPS_enum
  slr_VHAL_PDKeyAreaPTG_enum : BusSelector  OutputSignals=VHAL_PDKeyAreaPTG_enum
  slr_VHAL_PDKeyWelcome_enum : BusSelector  OutputSignals=VHAL_PDKeyWelcome_enum
  slr_VHAL_PDkeyShowIVI_enum : BusSelector  OutputSignals=VHAL_PDkeyShowIVI_enum
  slr_VHAL_PKeyMiss_flg : BusSelector  OutputSignals=VHAL_PKeyMiss_flg
  slr_VHAL_PKeyMode_enum : BusSelector  OutputSignals=VHAL_PKeyMode_enum
  slr_VHAL_PUIDLowPower_flg : BusSelector  OutputSignals=VHAL_PUIDLowPower_flg
  VINP_DKCKeyNumSta_enum : Outport
  VINP_DKCKeyTypeSta_enum : Outport  Port=2
  VINP_DKCPDkeyAreaRAPSSta_enum : Outport  Port=3
  VINP_DKCParkingModeCmd_enum : Outport  Port=4
  VINP_DKCReVehData_enum : Outport  Port=5
  VINP_PCommandToBCM_enum : Outport  Port=6
  VINP_PCommandToPTG_enum : Outport  Port=7
  VINP_PDKeyAreaLockUnlock_enum : Outport  Port=8
  VINP_PDKeyAreaPS_enum : Outport  Port=9
  VINP_PDKeyAreaPTG_enum : Outport  Port=10
  VINP_PDKeyWelcome_enum : Outport  Port=11
  VINP_PDkeyShowIVI_enum : Outport  Port=12
  VINP_PKeyMiss_flg : Outport  Port=13
  VINP_PKeyMode_enum : Outport  Port=14
  VINP_PUIDLowPower_flg : Outport  Port=15
  wires:
  BHAL_outputs/1 -> [BHAL_outputs]
  inp_CanValid_bus/1 -> [inp_CanValid_bus]
  [BHAL_outputs] -> slr_VHAL_DKCKeyNumSta_enum/1
  slr_VHAL_DKCKeyNumSta_enum/1 -> DKCKeyNumSta/1  "<VHAL_DKCKeyNumSta_enum>"
  True_VHAL_DKCKeyNumSta_enum/1 -> DKCKeyNumSta/2
  [inp_CanValid_bus] -> slr1_1/1
  slr1_1/1 -> DKCKeyNumSta/3  "<VINP_CANMsgValidDKC1_flg>"
  DKCKeyNumSta/1 -> VINP_DKCKeyNumSta_enum/1  "VINP_DKCKeyNumSta_enum"
  DKCKeyNumSta/2 -> Terminator_1/1
  [BHAL_outputs] -> slr_VHAL_DKCKeyTypeSta_enum/1
  slr_VHAL_DKCKeyTypeSta_enum/1 -> DKCKeyTypeSta/1  "<VHAL_DKCKeyTypeSta_enum>"
  True_VHAL_DKCKeyTypeSta_enum/1 -> DKCKeyTypeSta/2
  [inp_CanValid_bus] -> slr1_2/1
  slr1_2/1 -> DKCKeyTypeSta/3  "<VINP_CANMsgValidDKC1_flg>"
  DKCKeyTypeSta/1 -> VINP_DKCKeyTypeSta_enum/1  "VINP_DKCKeyTypeSta_enum"
  DKCKeyTypeSta/2 -> Terminator_2/1
  [BHAL_outputs] -> slr_VHAL_DKCPDkeyAreaRAPSSta_enum/1
  slr_VHAL_DKCPDkeyAreaRAPSSta_enum/1 -> DKCPDkeyAreaRAPSSta/1  "<VHAL_DKCPDkeyAreaRAPSSta_enum>"
  True_VHAL_DKCPDkeyAreaRAPSSta_enum/1 -> DKCPDkeyAreaRAPSSta/2
  [inp_CanValid_bus] -> slr1_3/1
  slr1_3/1 -> DKCPDkeyAreaRAPSSta/3  "<VINP_CANMsgValidDKC1_flg>"
  DKCPDkeyAreaRAPSSta/1 -> VINP_DKCPDkeyAreaRAPSSta_enum/1  "VINP_DKCPDkeyAreaRAPSSta_enum"
  DKCPDkeyAreaRAPSSta/2 -> Terminator_3/1
  [BHAL_outputs] -> slr_VHAL_DKCParkingModeCmd_enum/1
  slr_VHAL_DKCParkingModeCmd_enum/1 -> DKCParkingModeCmd/1  "<VHAL_DKCParkingModeCmd_enum>"
  True_VHAL_DKCParkingModeCmd_enum/1 -> DKCParkingModeCmd/2
  [inp_CanValid_bus] -> slr1_4/1
  slr1_4/1 -> DKCParkingModeCmd/3  "<VINP_CANMsgValidDKC1_flg>"
  DKCParkingModeCmd/1 -> VINP_DKCParkingModeCmd_enum/1  "VINP_DKCParkingModeCmd_enum"
  DKCParkingModeCmd/2 -> Terminator_4/1
  [BHAL_outputs] -> slr_VHAL_DKCReVehData_enum/1
  slr_VHAL_DKCReVehData_enum/1 -> DKCReVehData/1  "<VHAL_DKCReVehData_enum>"
  True_VHAL_DKCReVehData_enum/1 -> DKCReVehData/2
  [inp_CanValid_bus] -> slr1_5/1
  slr1_5/1 -> DKCReVehData/3  "<VINP_CANMsgValidDKC1_flg>"
  DKCReVehData/1 -> VINP_DKCReVehData_enum/1  "VINP_DKCReVehData_enum"
  DKCReVehData/2 -> Terminator_5/1
  [BHAL_outputs] -> slr_VHAL_PCommandToBCM_enum/1
  slr_VHAL_PCommandToBCM_enum/1 -> PCommandToBCM/1  "<VHAL_PCommandToBCM_enum>"
  True_VHAL_PCommandToBCM_enum/1 -> PCommandToBCM/2
  [inp_CanValid_bus] -> slr1_6/1
  slr1_6/1 -> PCommandToBCM/3  "<VINP_CANMsgValidDKC1_flg>"
  PCommandToBCM/1 -> VINP_PCommandToBCM_enum/1  "VINP_PCommandToBCM_enum"
  PCommandToBCM/2 -> Terminator_6/1
  [BHAL_outputs] -> slr_VHAL_PCommandToPTG_enum/1
  slr_VHAL_PCommandToPTG_enum/1 -> PCommandToPTG/1  "<VHAL_PCommandToPTG_enum>"
  True_VHAL_PCommandToPTG_enum/1 -> PCommandToPTG/2
  [inp_CanValid_bus] -> slr1_7/1
  slr1_7/1 -> PCommandToPTG/3  "<VINP_CANMsgValidDKC1_flg>"
  PCommandToPTG/1 -> VINP_PCommandToPTG_enum/1  "VINP_PCommandToPTG_enum"
  PCommandToPTG/2 -> Terminator_7/1
  [BHAL_outputs] -> slr_VHAL_PDKeyAreaLockUnlock_enum/1
  slr_VHAL_PDKeyAreaLockUnlock_enum/1 -> PDKeyAreaLockUnlock/1  "<VHAL_PDKeyAreaLockUnlock_enum>"
  True_VHAL_PDKeyAreaLockUnlock_enum/1 -> PDKeyAreaLockUnlock/2
  [inp_CanValid_bus] -> slr1_8/1
  slr1_8/1 -> PDKeyAreaLockUnlock/3  "<VINP_CANMsgValidDKC1_flg>"
  PDKeyAreaLockUnlock/1 -> VINP_PDKeyAreaLockUnlock_enum/1  "VINP_PDKeyAreaLockUnlock_enum"
  PDKeyAreaLockUnlock/2 -> Terminator_8/1
  [BHAL_outputs] -> slr_VHAL_PDKeyAreaPS_enum/1
  slr_VHAL_PDKeyAreaPS_enum/1 -> PDKeyAreaPS/1  "<VHAL_PDKeyAreaPS_enum>"
  True_VHAL_PDKeyAreaPS_enum/1 -> PDKeyAreaPS/2
  [inp_CanValid_bus] -> slr1_9/1
  slr1_9/1 -> PDKeyAreaPS/3  "<VINP_CANMsgValidDKC1_flg>"
  PDKeyAreaPS/1 -> VINP_PDKeyAreaPS_enum/1  "VINP_PDKeyAreaPS_enum"
  PDKeyAreaPS/2 -> Terminator_9/1
  [BHAL_outputs] -> slr_VHAL_PDKeyAreaPTG_enum/1
  slr_VHAL_PDKeyAreaPTG_enum/1 -> PDKeyAreaPTG/1  "<VHAL_PDKeyAreaPTG_enum>"
  True_VHAL_PDKeyAreaPTG_enum/1 -> PDKeyAreaPTG/2
  [inp_CanValid_bus] -> slr1_10/1
  slr1_10/1 -> PDKeyAreaPTG/3  "<VINP_CANMsgValidDKC1_flg>"
  PDKeyAreaPTG/1 -> VINP_PDKeyAreaPTG_enum/1  "VINP_PDKeyAreaPTG_enum"
  PDKeyAreaPTG/2 -> Terminator_10/1
  [BHAL_outputs] -> slr_VHAL_PDKeyWelcome_enum/1
  slr_VHAL_PDKeyWelcome_enum/1 -> PDKeyWelcome/1  "<VHAL_PDKeyWelcome_enum>"
  True_VHAL_PDKeyWelcome_enum/1 -> PDKeyWelcome/2
  [inp_CanValid_bus] -> slr1_11/1
  slr1_11/1 -> PDKeyWelcome/3  "<VINP_CANMsgValidDKC1_flg>"
  PDKeyWelcome/1 -> VINP_PDKeyWelcome_enum/1  "VINP_PDKeyWelcome_enum"
  PDKeyWelcome/2 -> Terminator_11/1
  [BHAL_outputs] -> slr_VHAL_PDkeyShowIVI_enum/1
  slr_VHAL_PDkeyShowIVI_enum/1 -> PDkeyShowIVI/1  "<VHAL_PDkeyShowIVI_enum>"
  True_VHAL_PDkeyShowIVI_enum/1 -> PDkeyShowIVI/2
  [inp_CanValid_bus] -> slr1_12/1
  slr1_12/1 -> PDkeyShowIVI/3  "<VINP_CANMsgValidDKC1_flg>"
  PDkeyShowIVI/1 -> VINP_PDkeyShowIVI_enum/1  "VINP_PDkeyShowIVI_enum"
  PDkeyShowIVI/2 -> Terminator_12/1
  [BHAL_outputs] -> slr_VHAL_PKeyMiss_flg/1
  slr_VHAL_PKeyMiss_flg/1 -> PKeyMiss/1  "<VHAL_PKeyMiss_flg>"
  True_VHAL_PKeyMiss_flg/1 -> PKeyMiss/2
  [inp_CanValid_bus] -> slr1_13/1
  slr1_13/1 -> PKeyMiss/3  "<VINP_CANMsgValidDKC1_flg>"
  PKeyMiss/1 -> VINP_PKeyMiss_flg/1  "VINP_PKeyMiss_flg"
  PKeyMiss/2 -> Terminator_13/1
  [BHAL_outputs] -> slr_VHAL_PKeyMode_enum/1
  slr_VHAL_PKeyMode_enum/1 -> PKeyMode/1  "<VHAL_PKeyMode_enum>"
  True_VHAL_PKeyMode_enum/1 -> PKeyMode/2
  [inp_CanValid_bus] -> slr1_14/1
  slr1_14/1 -> PKeyMode/3  "<VINP_CANMsgValidDKC1_flg>"
  PKeyMode/1 -> VINP_PKeyMode_enum/1  "VINP_PKeyMode_enum"
  PKeyMode/2 -> Terminator_14/1
  [BHAL_outputs] -> slr_VHAL_PUIDLowPower_flg/1
  slr_VHAL_PUIDLowPower_flg/1 -> PUIDLowPower/1  "<VHAL_PUIDLowPower_flg>"
  True_VHAL_PUIDLowPower_flg/1 -> PUIDLowPower/2
  [inp_CanValid_bus] -> slr1_15/1
  slr1_15/1 -> PUIDLowPower/3  "<VINP_CANMsgValidDKC1_flg>"
  PUIDLowPower/1 -> VINP_PUIDLowPower_flg/1  "VINP_PUIDLowPower_flg"
  PUIDLowPower/2 -> Terminator_15/1

== system inp/INP/CAN4/SignalCheck/DKC2 ==
  BHAL_outputs : Inport
  inp_CanValid_bus : Inport  Port=2
  EncryptionDATA063 : FVT_lib/inp/can_signal_template  SystemSampleTime=-1  VariantActivationTime=update diagram  Latency=0  AutoFrameSizeCalculation=off
      link override defval: Value=KINP_EncryptionDATA063_enum_defval
      link override ovrdflg: Value=KINP_EncryptionDATA063_enum_ovrdflg
      link override ovrdval: Value=KINP_EncryptionDATA063_enum_ovrdval
  EncryptionDATA64127 : FVT_lib/inp/can_signal_template  SystemSampleTime=-1  VariantActivationTime=update diagram  Latency=0  AutoFrameSizeCalculation=off
      link override defval: Value=KINP_EncryptionDATA64127_enum_defval
      link override ovrdflg: Value=KINP_EncryptionDATA64127_enum_ovrdflg
      link override ovrdval: Value=KINP_EncryptionDATA64127_enum_ovrdval
  RandomNumberX : FVT_lib/inp/can_signal_template  SystemSampleTime=-1  VariantActivationTime=update diagram  Latency=0  AutoFrameSizeCalculation=off
      link override defval: Value=KINP_RandomNumberX_enum_defval
      link override ovrdflg: Value=KINP_RandomNumberX_enum_ovrdflg
      link override ovrdval: Value=KINP_RandomNumberX_enum_ovrdval
  Terminator_1 : Terminator
  Terminator_2 : Terminator
  Terminator_3 : Terminator
  True_VHAL_EncryptionDATA063_enum : Constant  Value=TRUE  OutDataTypeStr=boolean
  True_VHAL_EncryptionDATA64127_enum : Constant  Value=TRUE  OutDataTypeStr=boolean
  True_VHAL_RandomNumberX_enum : Constant  Value=TRUE  OutDataTypeStr=boolean
  slr1_1 : BusSelector  OutputSignals=VINP_CANMsgValidDKC2_flg
  slr1_2 : BusSelector  OutputSignals=VINP_CANMsgValidDKC2_flg
  slr1_3 : BusSelector  OutputSignals=VINP_CANMsgValidDKC2_flg
  slr_VHAL_EncryptionDATA063_enum : BusSelector  OutputSignals=VHAL_EncryptionDATA063_enum
  slr_VHAL_EncryptionDATA64127_enum : BusSelector  OutputSignals=VHAL_EncryptionDATA64127_enum
  slr_VHAL_RandomNumberX_enum : BusSelector  OutputSignals=VHAL_RandomNumberX_enum
  VINP_EncryptionDATA063_enum : Outport
  VINP_EncryptionDATA64127_enum : Outport  Port=2
  VINP_RandomNumberX_enum : Outport  Port=3
  wires:
  BHAL_outputs/1 -> [BHAL_outputs]
  inp_CanValid_bus/1 -> [inp_CanValid_bus]
  [BHAL_outputs] -> slr_VHAL_EncryptionDATA063_enum/1
  slr_VHAL_EncryptionDATA063_enum/1 -> EncryptionDATA063/1  "<VHAL_EncryptionDATA063_enum>"
  True_VHAL_EncryptionDATA063_enum/1 -> EncryptionDATA063/2
  [inp_CanValid_bus] -> slr1_1/1
  slr1_1/1 -> EncryptionDATA063/3  "<VINP_CANMsgValidDKC2_flg>"
  EncryptionDATA063/1 -> VINP_EncryptionDATA063_enum/1  "VINP_EncryptionDATA063_enum"
  EncryptionDATA063/2 -> Terminator_1/1
  [BHAL_outputs] -> slr_VHAL_EncryptionDATA64127_enum/1
  slr_VHAL_EncryptionDATA64127_enum/1 -> EncryptionDATA64127/1  "<VHAL_EncryptionDATA64127_enum>"
  True_VHAL_EncryptionDATA64127_enum/1 -> EncryptionDATA64127/2
  [inp_CanValid_bus] -> slr1_2/1
  slr1_2/1 -> EncryptionDATA64127/3  "<VINP_CANMsgValidDKC2_flg>"
  EncryptionDATA64127/1 -> VINP_EncryptionDATA64127_enum/1  "VINP_EncryptionDATA64127_enum"
  EncryptionDATA64127/2 -> Terminator_2/1
  [BHAL_outputs] -> slr_VHAL_RandomNumberX_enum/1
  slr_VHAL_RandomNumberX_enum/1 -> RandomNumberX/1  "<VHAL_RandomNumberX_enum>"
  True_VHAL_RandomNumberX_enum/1 -> RandomNumberX/2
  [inp_CanValid_bus] -> slr1_3/1
  slr1_3/1 -> RandomNumberX/3  "<VINP_CANMsgValidDKC2_flg>"
  RandomNumberX/1 -> VINP_RandomNumberX_enum/1  "VINP_RandomNumberX_enum"
  RandomNumberX/2 -> Terminator_3/1
